simulink model "controller_sdfp_host"  (Simulink 7.3)
settings: Solver=ode45  StartTime=0.0  StopTime=2  RelTol=1e-3
values from neighbouring files (symbols this model uses):
  d = 16    [one_bit_control.m]
  delay_shift1 = -k_preint    (= 0)    [one_bit_control.m]
  delay_shift2 = -k_preint    (= 0)    [one_bit_control.m]
  delay_shift3 = -k_preint    (= 0)    [one_bit_control.m]
  fixpt_adder_in_bitwidth = w    (= 24)    [one_bit_control.m]
  fixpt_adder_in_position = d    (= 16)    [one_bit_control.m]
  fixpt_adder_out_bitwidth = w    (= 24)    [one_bit_control.m]
  fixpt_adder_out_position = d    (= 16)    [one_bit_control.m]
  fixpt_gain_bitwidth = w    (= 24)    [one_bit_control.m]
  fixpt_gain_position = d    (= 16)    [one_bit_control.m]
  k = 2^k_bitshift    (= 0.000244140625)    [one_bit_control.m]
  p0 = 1326*T^3*k^-3    [one_bit_control.m]
  p1 = 9397*T^2*k^-2    [one_bit_control.m]
  p2 = 262.3*T*k^-1    [one_bit_control.m]
  p3 = 16.65    [one_bit_control.m]
  postint_gain1 = k_postint    (= -12)    [one_bit_control.m]
  postint_gain2 = k_postint    (= -12)    [one_bit_control.m]
  postint_gain3 = k_postint    (= -12)    [one_bit_control.m]
  preint_gain1 = k_preint    (= 0)    [one_bit_control.m]
  preint_gain2 = k_preint    (= 0)    [one_bit_control.m]
  preint_gain3 = k_preint    (= 0)    [one_bit_control.m]
  q0 = 0*T^3*k^-3    [one_bit_control.m]
  q1 = 400.8*T^2*k^-2    [one_bit_control.m]
  q2 = 33.2*T*k^-1    [one_bit_control.m]
  T = ts    [one_bit_control.m]
  ts = 1/Fs    [one_bit_control.m]
  w = 24    [one_bit_control.m]
libraries: simulink x16, commnoisgen2 x1, cstblocks x1
(part 1 of 2)
settings Model: Creator=Joseph Poverelli  LastModifiedBy=kunal
settings OptimizationCC: InitFltsAndDblsToZero=on

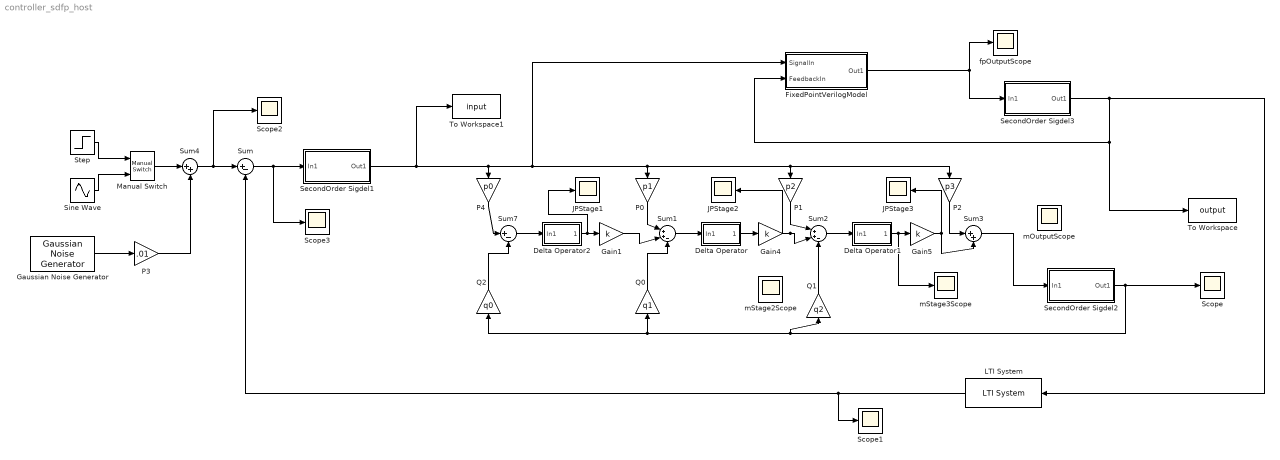
== system controller_sdfp_host ==
  Delta Operator : Subsystem
  Delta Operator1 : Subsystem
  Delta Operator2 : Subsystem
  FixedPointVerilogModel : Subsystem
  Gain1 : Gain  Gain=k  ParameterDataType=sfix(16)  ParameterScaling=2^0  OutDataType=fixdt(1,w,d)  RndMeth=Nearest
  Gain4 : Gain  Gain=k  ParameterDataType=sfix(16)  ParameterScaling=2^0  OutDataType=fixdt(1,w,d)  RndMeth=Nearest
  Gain5 : Gain  Gain=k  ParameterDataType=sfix(16)  ParameterScaling=2^0  OutDataType=fixdt(1,w,d)  RndMeth=Nearest
  Gaussian Noise Generator : commnoisgen2/Gaussian Noise Generator  SystemSampleTime=-1  m=0  d=1  s=41  Ts=T  frameBased=off  sampPerFrame=1  orient=off  outDataType=double
  JPStage1 : Scope
      settings: YMin=-30  YMax=30  SaveName=ScopeData12
  JPStage2 : Scope
      settings: YMin=-0.03  YMax=0.11  SaveName=ScopeData5
  JPStage3 : Scope
      settings: YMin=-0.35  YMax=0.25  SaveName=ScopeData9
  LTI System : cstblocks/LTI System  SystemSampleTime=-1  sys=P  IC=[]
  Manual Switch : simulink/Signal Routing/Manual Switch  SystemSampleTime=-1  sw=0  action=0  varsize=off
  P0 : Gain  Gain=p1  ParameterDataType=sfix(16)  ParameterScaling=2^0  OutDataType=sfix(16)  OutScaling=2^0
  P1 : Gain  Gain=p2  ParameterDataType=sfix(16)  ParameterScaling=2^0  OutDataType=sfix(16)  OutScaling=2^0
  P2 : Gain  Gain=p3  ParameterDataType=sfix(16)  ParameterScaling=2^0  OutDataType=sfix(16)  OutScaling=2^0
  P3 : Gain  Gain=.01  ParameterDataType=sfix(16)  ParameterScaling=2^0  OutDataType=sfix(16)  OutScaling=2^0
  P4 : Gain  Gain=p0  ParameterDataType=sfix(16)  ParameterScaling=2^0  OutDataType=sfix(16)  OutScaling=2^0
  Q0 : Gain  Gain=q1  ParameterDataType=sfix(16)  ParameterScaling=2^0  OutDataType=sfix(16)  OutScaling=2^0
  Q1 : Gain  Gain=q2  ParameterDataType=sfix(16)  ParameterScaling=2^0  OutDataType=sfix(16)  OutScaling=2^0
  Q2 : Gain  Gain=q0  ParameterDataType=sfix(16)  ParameterScaling=2^0  OutDataType=sfix(16)  OutScaling=2^0
  Scope{,1..3} (4 alike) : Scope
      Scope settings: YMin=-1  YMax=1  SaveName=Y  DataFormat=Structure  SampleInput=on  SampleTime=ts
      Scope1 settings: YMin=-0.10575  YMax=-0.1035  SaveName=plant_output  DataFormat=Structure  SampleInput=on  SampleTime=ts
      Scope2 settings: YMin=-0.04  YMax=0.07  SaveName=in  DataFormat=Structure  SampleInput=on  SampleTime=ts
      Scope3 settings: YMin=0.06375  YMax=0.06575  SaveName=error  DataFormat=Array  SampleInput=on  SampleTime=ts
  SecondOrder Sigdel1 : Subsystem
  SecondOrder Sigdel2 : Subsystem
  SecondOrder Sigdel3 : Subsystem
  Sine Wave : Sin  Amplitude=.03  Bias=0  Frequency=2*pi*20  Phase=0  Samples=10  SampleTime=0  Offset=0
  Step : Step  After=.1  SampleTime=ts
  Sum : Sum  Inputs=|+-  OutDataType=sfix(16)  OutScaling=2^0
  Sum1 : Sum  Inputs=|++-  OutDataType=fixdt(1,w,d)  RndMeth=Nearest
  Sum2 : Sum  Inputs=|++-  OutDataType=fixdt(1,w,d)  RndMeth=Nearest
  Sum3 : Sum  Inputs=|++  OutMin=[-p2]  OutMax=[p2]  OutDataType=fixdt(1,w,d)  RndMeth=Nearest  SaturateOnIntegerOverflow=on
  Sum4 : Sum  Inputs=|++  OutDataType=sfix(16)  OutScaling=2^0
  Sum7 : Sum  Inputs=|+-  OutDataType=fixdt(1,w,d)  RndMeth=Nearest
  To Workspace : ToWorkspace  VariableName=output  SampleTime=-1  SaveFormat=Array
  To Workspace1 : ToWorkspace  VariableName=input  SampleTime=-1  SaveFormat=Array
  fpOutputScope : Scope
      settings: YMin=-9.97  YMax=-9.8  SaveName=c_output1  DataFormat=Structure  SampleInput=on  SampleTime=ts
  mOutputScope : Scope
      settings: YMin=-9.97  YMax=-9.8  SaveName=c_output  DataFormat=Structure  SampleInput=on  SampleTime=ts
  mStage2Scope : Scope
      settings: YMin=-0.175  YMax=0.025  SaveName=delta3  DataFormat=Array  SampleInput=on  SampleTime=ts
  mStage3Scope : Scope
      settings: YMin=-0.225  YMax=0.025  SaveName=delta  DataFormat=Array  SampleInput=on  SampleTime=ts
  wires:
  Sum/1 -> SecondOrder Sigdel1/1(In1), Scope3/1
  LTI System/1 -> Sum/2, Scope1/1
  SecondOrder Sigdel1/1(Out1) -> P4/1, P0/1, P1/1, P2/1, FixedPointVerilogModel/1(SignalIn), To Workspace1/1
  Sum3/1 -> SecondOrder Sigdel2/1(In1)
  P0/1 -> Sum1/1
  Q1/1 -> Sum2/3
  P1/1 -> Sum2/1
  P2/1 -> Sum3/1
  Gain5/1 -> Sum3/2, JPStage3/1
  SecondOrder Sigdel2/1(Out1) -> Scope/1, Q1/1, Q0/1, Q2/1
  Delta Operator/1(Out1) -> Gain4/1
  Sum1/1 -> Delta Operator/1(In1)
  Sum2/1 -> Delta Operator1/1(In1)
  Delta Operator1/1(Out1) -> Gain5/1, mStage3Scope/1
  Manual Switch/1 -> Sum4/1
  Gaussian Noise Generator/1 -> P3/1
  Sum4/1 -> Sum/1, Scope2/1
  P3/1 -> Sum4/2
  Sine Wave/1 -> Manual Switch/2
  Step/1 -> Manual Switch/1
  P4/1 -> Sum7/1
  Q2/1 -> Sum7/2
  Delta Operator2/1(Out1) -> Gain1/1, JPStage1/1
  Sum7/1 -> Delta Operator2/1(In1)
  Q0/1 -> Sum1/3
  Gain1/1 -> Sum1/2
  Gain4/1 -> Sum2/2, JPStage2/1
  FixedPointVerilogModel/1(Out1) -> fpOutputScope/1, SecondOrder Sigdel3/1(In1)
  SecondOrder Sigdel3/1(Out1) -> LTI System/1, FixedPointVerilogModel/2(FeedbackIn), To Workspace/1

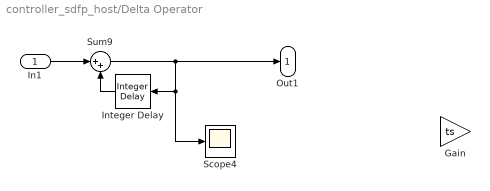
== system controller_sdfp_host/Delta Operator ==
  In1 : Inport  OutDataType=sfix(16)  OutScaling=2^0
  Gain : Gain  Gain=ts  ParameterDataType=sfix(16)  ParameterScaling=2^0  OutDataType=fixdt(1,w,d)  RndMeth=Nearest
  Integer Delay : simulink/Discrete/Integer Delay  vinit=0.0  samptime=-1  NumDelays=1
  Scope4 : Scope
      settings: YMin=-10  YMax=10  SaveName=delta1  DataFormat=Array  SampleInput=on  SampleTime=ts
  Sum9 : Sum  Inputs=|++  OutDataType=fixdt(1,w,d)  RndMeth=Nearest  SampleTime=ts
  Out1 : Outport  OutDataType=sfix(16)  OutScaling=2^0
  wires:
  In1/1 -> Sum9/1
  Sum9/1 -> Integer Delay/1, Scope4/1, Out1/1
  Integer Delay/1 -> Sum9/2

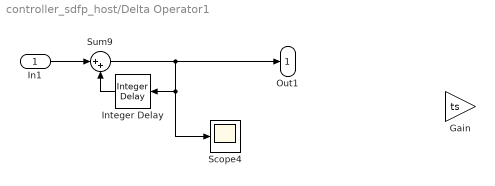
== system controller_sdfp_host/Delta Operator1 ==
  In1 : Inport  OutDataType=sfix(16)  OutScaling=2^0
  Gain : Gain  Gain=ts  ParameterDataType=sfix(16)  ParameterScaling=2^0  OutDataType=fixdt(1,w,d)  RndMeth=Nearest
  Integer Delay : simulink/Discrete/Integer Delay  vinit=0.0  samptime=-1  NumDelays=1
  Scope4 : Scope
      settings: YMin=-10  YMax=10  SaveName=delta2  DataFormat=Array  SampleInput=on  SampleTime=ts
  Sum9 : Sum  Inputs=|++  OutDataType=fixdt(1,w,d)  RndMeth=Nearest  SampleTime=ts
  Out1 : Outport  OutDataType=sfix(16)  OutScaling=2^0
  wires:
  In1/1 -> Sum9/1
  Sum9/1 -> Integer Delay/1, Scope4/1, Out1/1
  Integer Delay/1 -> Sum9/2

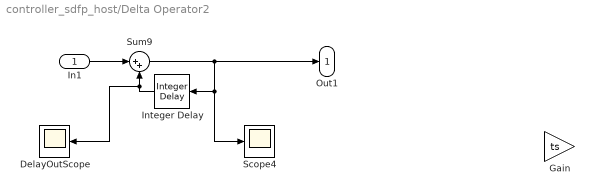
== system controller_sdfp_host/Delta Operator2 ==
  In1 : Inport  OutDataType=sfix(16)  OutScaling=2^0
  DelayOutScope : Scope
      settings: YMin=-900  YMax=700  SaveName=delta4  DataFormat=Array  SampleInput=on  SampleTime=ts
  Gain : Gain  Gain=ts  ParameterDataType=sfix(16)  ParameterScaling=2^0  OutDataType=fixdt(1,w,d)  RndMeth=Nearest
  Integer Delay : simulink/Discrete/Integer Delay  vinit=0.0  samptime=-1  NumDelays=1
  Scope4 : Scope
      settings: TimeRange=0.5  YMin=0.038443  YMax=0.0424896  SaveName=delta43  DataFormat=Array  SampleInput=on  SampleTime=ts
  Sum9 : Sum  Inputs=|++  OutDataType=fixdt(1,w,d)  RndMeth=Nearest  SampleTime=ts
  Out1 : Outport  OutDataType=sfix(16)  OutScaling=2^0
  wires:
  In1/1 -> Sum9/1
  Sum9/1 -> Integer Delay/1, Scope4/1, Out1/1
  Integer Delay/1 -> Sum9/2, DelayOutScope/1

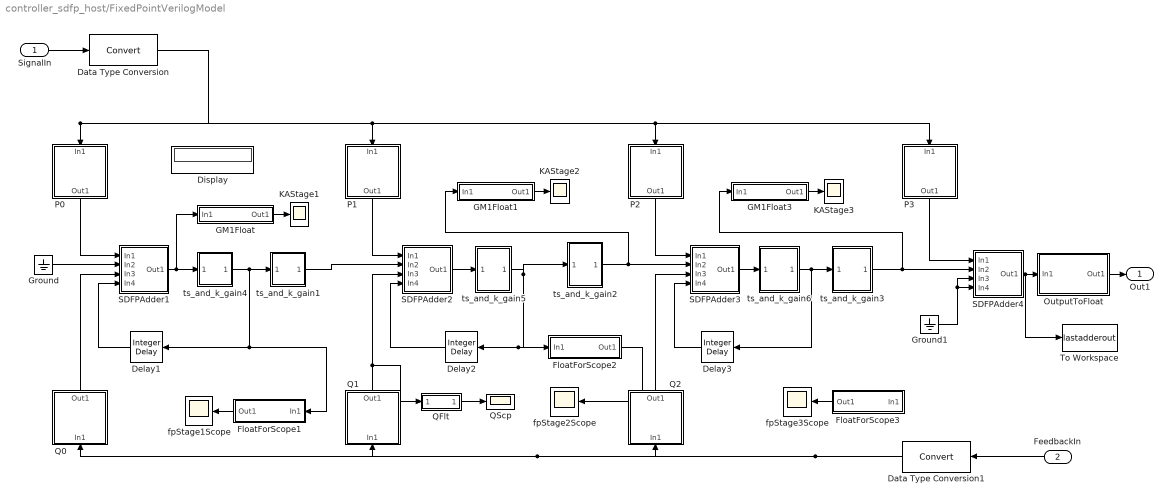
== system controller_sdfp_host/FixedPointVerilogModel ==
  SignalIn : Inport  OutDataType=fixdt(1, 16)  OutScaling=2^0
  FeedbackIn : Inport  Port=2  OutDataType=fixdt(1, 16)  OutScaling=2^0
  Data Type Conversion : DataTypeConversion  OutDataType=fixdt(1, 16)  OutScaling=2^0
  Data Type Conversion1 : DataTypeConversion  OutDataType=fixdt(1, 16)  OutScaling=2^0
  Delay1 : simulink/Discrete/Integer Delay  vinit=0.0  samptime=-1  NumDelays=1
  Delay2 : simulink/Discrete/Integer Delay  vinit=0.0  samptime=-1  NumDelays=1
  Delay3 : simulink/Discrete/Integer Delay  vinit=0.0  samptime=-1  NumDelays=1
  Display : Display
      settings: Format=hex (Stored Integer)
  FloatForScope1 : Subsystem  mask{bitwidth=fixpt_adder_out_bitwidth, fp_position=fixpt_adder_out_position}
      mask prompts: bitwidth "Input Bitwidth"; fp_position "Input Point Position"
      mask Display: disp('Fixed -> Float');
  FloatForScope2 : Subsystem  mask{bitwidth=fixpt_adder_out_bitwidth, fp_position=fixpt_adder_out_position}
      mask prompts: bitwidth "Input Bitwidth"; fp_position "Input Point Position"
      mask Display: disp('Fixed -> Float');
  FloatForScope3 : Subsystem  mask{bitwidth=fixpt_adder_out_bitwidth, fp_position=fixpt_adder_out_position}
      mask prompts: bitwidth "Input Bitwidth"; fp_position "Input Point Position"
      mask Display: disp('Fixed -> Float');
  GM1Float : Subsystem  mask{bitwidth=fixpt_gain_bitwidth, fp_position=fixpt_gain_position}
      mask prompts: bitwidth "Input Bitwidth"; fp_position "Input Point Position"
      mask Display: disp('Fixed -> Float');
  GM1Float1 : Subsystem  mask{bitwidth=fixpt_gain_bitwidth, fp_position=fixpt_gain_position}
      mask prompts: bitwidth "Input Bitwidth"; fp_position "Input Point Position"
      mask Display: disp('Fixed -> Float');
  GM1Float3 : Subsystem  mask{bitwidth=fixpt_gain_bitwidth, fp_position=fixpt_gain_position}
      mask prompts: bitwidth "Input Bitwidth"; fp_position "Input Point Position"
      mask Display: disp('Fixed -> Float');
  Ground : Ground
  Ground1 : Ground
  KAStage1 : Scope
      settings: YMin=-1  YMax=1  SaveName=ScopeData6
  KAStage2 : Scope
      settings: YMin=-0.035  YMax=0.055  SaveName=ScopeData3
  KAStage3 : Scope
      settings: YMin=-0.0007  YMax=0.0009  SaveName=ScopeData14
  OutputToFloat : Subsystem  mask{bitwidth=fixpt_adder_out_bitwidth, fp_position=fixpt_adder_out_position}
      mask prompts: bitwidth "Input Bitwidth"; fp_position "Input Point Position"
      mask Display: disp('Fixed -> Float');
  P0 : Subsystem  mask{gain=p0, bitwidth=fixpt_gain_bitwidth, fp_position=fixpt_gain_position}
      mask prompts: bitwidth "Output Bitwidth"; fp_position "Output Point Position"
      mask Display: plot([0.2 0.9 0.2 0.2],[0 .5 1 0]);disp('GainMux')
  P1 : Subsystem  mask{gain=p1, bitwidth=fixpt_gain_bitwidth, fp_position=fixpt_gain_position}
      mask prompts: bitwidth "Output Bitwidth"; fp_position "Output Point Position"
      mask Display: plot([0.2 0.9 0.2 0.2],[0 .5 1 0]);disp('GainMux')
  P2 : Subsystem  mask{gain=p2, bitwidth=fixpt_gain_bitwidth, fp_position=fixpt_gain_position}
      mask prompts: bitwidth "Output Bitwidth"; fp_position "Output Point Position"
      mask Display: plot([0.2 0.9 0.2 0.2],[0 .5 1 0]);disp('GainMux')
  P3 : Subsystem  mask{gain=p3, bitwidth=fixpt_gain_bitwidth, fp_position=fixpt_gain_position}
      mask prompts: bitwidth "Output Bitwidth"; fp_position "Output Point Position"
      mask Display: plot([0.2 0.9 0.2 0.2],[0 .5 1 0]);disp('GainMux')
  Q0 : Subsystem  mask{gain=q0, bitwidth=fixpt_gain_bitwidth, fp_position=fixpt_gain_position}
      mask prompts: bitwidth "Output Bitwidth"; fp_position "Output Point Position"
      mask Display: plot([0.2 0.9 0.2 0.2],[0 .5 1 0]);disp('GainMux')
  Q1 : Subsystem  mask{gain=q1, bitwidth=fixpt_gain_bitwidth, fp_position=fixpt_gain_position}
      mask prompts: bitwidth "Output Bitwidth"; fp_position "Output Point Position"
      mask Display: plot([0.2 0.9 0.2 0.2],[0 .5 1 0]);disp('GainMux')
  Q2 : Subsystem  mask{gain=q2, bitwidth=fixpt_gain_bitwidth, fp_position=fixpt_gain_position}
      mask prompts: bitwidth "Output Bitwidth"; fp_position "Output Point Position"
      mask Display: plot([0.2 0.9 0.2 0.2],[0 .5 1 0]);disp('GainMux')
  QFlt : Subsystem  mask{bitwidth=fixpt_gain_bitwidth, fp_position=fixpt_gain_position}
      mask prompts: bitwidth "Input Bitwidth"; fp_position "Input Point Position"
      mask Display: disp('Fixed -> Float');
  QScp : Scope
      settings: SaveName=ScopeData11
  SDFPAdder1 : Subsystem  mask{in_bitwidth=fixpt_adder_in_bitwidth, in_fp_position=fixpt_adder_in_position, out_bitwidth=fixpt_adder_out_bitwidth, out_fp_position=fixpt_adder_out_position, in1_shift=0, in2_shift=0, in3_shift=0, in4_shift=delay_shift1}
      mask prompts: in_bitwidth "Input Bitwidth"; in_fp_position "Input Point Position"; out_bitwidth "Output Bitwidth"; out_fp_position "Output Point Position"; in1_shift "Input1 Pre-Shift"; in2_shift "Input2 Pre-Shift"; in3_shift "Input3 Pre-Shift"; in4_shift "Input4 Pre-Shift"
      mask Display: disp(['+\nSDFP'])
  SDFPAdder2 : Subsystem  mask{in_bitwidth=fixpt_adder_in_bitwidth, in_fp_position=fixpt_adder_in_position, out_bitwidth=fixpt_adder_out_bitwidth, out_fp_position=fixpt_adder_out_position, in1_shift=0, in2_shift=0, in3_shift=0, in4_shift=delay_shift2}
      mask prompts: in_bitwidth "Input Bitwidth"; in_fp_position "Input Point Position"; out_bitwidth "Output Bitwidth"; out_fp_position "Output Point Position"; in1_shift "Input1 Pre-Shift"; in2_shift "Input2 Pre-Shift"; in3_shift "Input3 Pre-Shift"; in4_shift "Input4 Pre-Shift"
      mask Display: disp(['+\nSDFP'])
  SDFPAdder3 : Subsystem  mask{in_bitwidth=fixpt_adder_in_bitwidth, in_fp_position=fixpt_adder_in_position, out_bitwidth=fixpt_adder_out_bitwidth, out_fp_position=fixpt_adder_out_position, in1_shift=0, in2_shift=0, in3_shift=0, in4_shift=delay_shift3}
      mask prompts: in_bitwidth "Input Bitwidth"; in_fp_position "Input Point Position"; out_bitwidth "Output Bitwidth"; out_fp_position "Output Point Position"; in1_shift "Input1 Pre-Shift"; in2_shift "Input2 Pre-Shift"; in3_shift "Input3 Pre-Shift"; in4_shift "Input4 Pre-Shift"
      mask Display: disp(['+\nSDFP'])
  SDFPAdder4 : Subsystem  mask{in_bitwidth=fixpt_adder_in_bitwidth, in_fp_position=fixpt_adder_in_position, out_bitwidth=fixpt_adder_out_bitwidth, out_fp_position=fixpt_adder_out_position, in1_shift=0, in2_shift=0, in3_shift=0, in4_shift=0}
      mask prompts: in_bitwidth "Input Bitwidth"; in_fp_position "Input Point Position"; out_bitwidth "Output Bitwidth"; out_fp_position "Output Point Position"; in1_shift "Input1 Pre-Shift"; in2_shift "Input2 Pre-Shift"; in3_shift "Input3 Pre-Shift"; in4_shift "Input4 Pre-Shift"
      mask Display: disp(['+\nSDFP'])
  To Workspace : ToWorkspace  VariableName=lastadderout  SampleTime=-1  SaveFormat=Array
  fpStage1Scope : Scope
      settings: YMin=-800  YMax=700
  fpStage2Scope : Scope
      settings: YMin=0  YMax=275
  fpStage3Scope : Scope
      settings: YMin=0  YMax=275  SaveName=ScopeData2
  ts_and_k_gain1 : Subsystem  mask{shift_amount=postint_gain1}
      mask init:
      | if(shift_amount > 0)
      |     dispval=sprintf('<< %d',shift_amount);
      | else
      |     dispval=sprintf('>> %d',-shift_amount);
      | end
      mask Display: disp(dispval);
  ts_and_k_gain2 : Subsystem  mask{shift_amount=postint_gain2}
      mask init:
      | if(shift_amount > 0)
      |     dispval=sprintf('<< %d',shift_amount);
      | else
      |     dispval=sprintf('>> %d',-shift_amount);
      | end
      mask Display: disp(dispval);
  ts_and_k_gain3 : Subsystem  mask{shift_amount=postint_gain3}
      mask init:
      | if(shift_amount > 0)
      |     dispval=sprintf('<< %d',shift_amount);
      | else
      |     dispval=sprintf('>> %d',-shift_amount);
      | end
      mask Display: disp(dispval);
  ts_and_k_gain4 : Subsystem  mask{shift_amount=preint_gain1}
      mask init:
      | if(shift_amount > 0)
      |     dispval=sprintf('<< %d',shift_amount);
      | else
      |     dispval=sprintf('>> %d',-shift_amount);
      | end
      mask Display: disp(dispval);
  ts_and_k_gain5 : Subsystem  mask{shift_amount=preint_gain2}
      mask init:
      | if(shift_amount > 0)
      |     dispval=sprintf('<< %d',shift_amount);
      | else
      |     dispval=sprintf('>> %d',-shift_amount);
      | end
      mask Display: disp(dispval);
  ts_and_k_gain6 : Subsystem  mask{shift_amount=preint_gain3}
      mask init:
      | if(shift_amount > 0)
      |     dispval=sprintf('<< %d',shift_amount);
      | else
      |     dispval=sprintf('>> %d',-shift_amount);
      | end
      mask Display: disp(dispval);
  Out1 : Outport  OutDataType=fixdt(1, 16)  OutScaling=2^0
  wires:
  P0/1(Out1) -> SDFPAdder1/1(In1)
  Ground/1 -> SDFPAdder1/2(In2)
  Delay1/1 -> SDFPAdder1/4(In4)
  Q0/1(Out1) -> SDFPAdder1/3(In3)
  P1/1(Out1) -> SDFPAdder2/1(In1)
  Delay2/1 -> SDFPAdder2/4(In4)
  Q1/1(Out1) -> QFlt/1(In1), SDFPAdder2/3(In3)
  SDFPAdder2/1(Out1) -> ts_and_k_gain5/1(In1)
  ts_and_k_gain1/1(Out1) -> SDFPAdder2/2(In2)
  P2/1(Out1) -> SDFPAdder3/1(In1)
  Delay3/1 -> SDFPAdder3/4(In4)
  Q2/1(Out1) -> SDFPAdder3/3(In3)
  ts_and_k_gain2/1(Out1) -> SDFPAdder3/2(In2), GM1Float1/1(In1)
  FeedbackIn/1 -> Data Type Conversion1/1
  ts_and_k_gain3/1(Out1) -> SDFPAdder4/2(In2), GM1Float3/1(In1)
  P3/1(Out1) -> SDFPAdder4/1(In1)
  SDFPAdder4/1(Out1) -> OutputToFloat/1(In1), To Workspace/1
  SignalIn/1 -> Data Type Conversion/1
  Data Type Conversion/1 -> P0/1(In1), P1/1(In1), P2/1(In1), P3/1(In1)
  Data Type Conversion1/1 -> Q2/1(In1), Q1/1(In1), Q0/1(In1)
  FloatForScope2/1(Out1) -> fpStage2Scope/1
  OutputToFloat/1(Out1) -> Out1/1
  QFlt/1(Out1) -> QScp/1
  GM1Float/1(Out1) -> KAStage1/1
  Ground1/1 -> SDFPAdder4/3(In3), SDFPAdder4/4(In4)
  FloatForScope1/1(Out1) -> fpStage1Scope/1
  SDFPAdder1/1(Out1) -> ts_and_k_gain4/1(In1), GM1Float/1(In1)
  ts_and_k_gain5/1(Out1) -> Delay2/1, FloatForScope2/1(In1), ts_and_k_gain2/1(In1)
  FloatForScope3/1(Out1) -> fpStage3Scope/1
  SDFPAdder3/1(Out1) -> ts_and_k_gain6/1(In1)
  ts_and_k_gain6/1(Out1) -> ts_and_k_gain3/1(In1), Delay3/1
  ts_and_k_gain4/1(Out1) -> ts_and_k_gain1/1(In1), Delay1/1, FloatForScope1/1(In1)
  GM1Float1/1(Out1) -> KAStage2/1
  GM1Float3/1(Out1) -> KAStage3/1

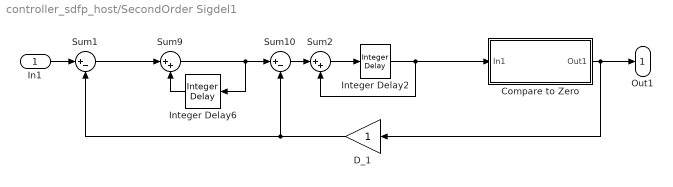
== system controller_sdfp_host/SecondOrder Sigdel1 ==
  In1 : Inport  OutDataType=sfix(16)  OutScaling=2^0
  Compare to Zero : Subsystem
  D_1 : Gain  ParameterDataType=sfix(16)  ParameterScaling=2^0  OutDataType=sfix(16)  OutScaling=2^0  SampleTime=ts
  Integer Delay2 : simulink/Discrete/Integer Delay  vinit=0.0  samptime=-1  NumDelays=1
  Integer Delay6 : simulink/Discrete/Integer Delay  vinit=0.0  samptime=-1  NumDelays=1
  Sum1 : Sum  Inputs=|+-  OutDataType=sfix(16)  OutScaling=2^0  SampleTime=ts
  Sum10 : Sum  Inputs=|+-  OutDataType=sfix(16)  OutScaling=2^0
  Sum2 : Sum  Inputs=|++  OutDataType=sfix(16)  OutScaling=2^0
  Sum9 : Sum  Inputs=|++  OutDataType=sfix(16)  OutScaling=2^0  SampleTime=ts
  Out1 : Outport  OutDataType=sfix(16)  OutScaling=2^0
  wires:
  Sum1/1 -> Sum9/1
  In1/1 -> Sum1/1
  Compare to Zero/1(Out1) -> D_1/1, Out1/1
  Sum2/1 -> Integer Delay2/1
  Integer Delay2/1 -> Sum2/2, Compare to Zero/1(In1)
  Sum9/1 -> Integer Delay6/1, Sum10/1
  Integer Delay6/1 -> Sum9/2
  Sum10/1 -> Sum2/1
  D_1/1 -> Sum1/2, Sum10/2

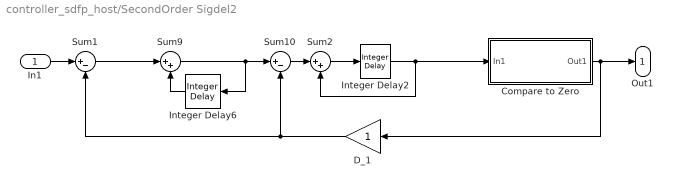
== system controller_sdfp_host/SecondOrder Sigdel2 ==
  In1 : Inport  OutDataType=sfix(16)  OutScaling=2^0
  Compare to Zero : Subsystem
  D_1 : Gain  ParameterDataType=sfix(16)  ParameterScaling=2^0  OutDataType=sfix(16)  OutScaling=2^0  SampleTime=ts
  Integer Delay2 : simulink/Discrete/Integer Delay  vinit=0.0  samptime=-1  NumDelays=1
  Integer Delay6 : simulink/Discrete/Integer Delay  vinit=0.0  samptime=-1  NumDelays=1
  Sum1 : Sum  Inputs=|+-  OutDataType=sfix(16)  OutScaling=2^0  SampleTime=ts
  Sum10 : Sum  Inputs=|+-  OutDataType=sfix(16)  OutScaling=2^0
  Sum2 : Sum  Inputs=|++  OutDataType=sfix(16)  OutScaling=2^0
  Sum9 : Sum  Inputs=|++  OutDataType=sfix(16)  OutScaling=2^0  SampleTime=ts
  Out1 : Outport  OutDataType=sfix(16)  OutScaling=2^0
  wires:
  Sum1/1 -> Sum9/1
  In1/1 -> Sum1/1
  Compare to Zero/1(Out1) -> D_1/1, Out1/1
  Sum2/1 -> Integer Delay2/1
  Integer Delay2/1 -> Sum2/2, Compare to Zero/1(In1)
  Sum9/1 -> Integer Delay6/1, Sum10/1
  Integer Delay6/1 -> Sum9/2
  Sum10/1 -> Sum2/1
  D_1/1 -> Sum1/2, Sum10/2

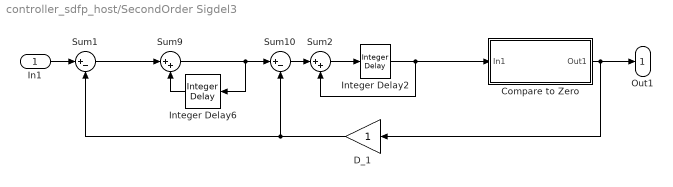
== system controller_sdfp_host/SecondOrder Sigdel3 ==
  In1 : Inport  OutDataType=sfix(16)  OutScaling=2^0
  Compare to Zero : Subsystem
  D_1 : Gain  ParameterDataType=sfix(16)  ParameterScaling=2^0  OutDataType=sfix(16)  OutScaling=2^0  SampleTime=ts
  Integer Delay2 : simulink/Discrete/Integer Delay  vinit=0.0  samptime=-1  NumDelays=1
  Integer Delay6 : simulink/Discrete/Integer Delay  vinit=0.0  samptime=-1  NumDelays=1
  Sum1 : Sum  Inputs=|+-  OutDataType=sfix(16)  OutScaling=2^0  SampleTime=ts
  Sum10 : Sum  Inputs=|+-  OutDataType=sfix(16)  OutScaling=2^0
  Sum2 : Sum  Inputs=|++  OutDataType=sfix(16)  OutScaling=2^0
  Sum9 : Sum  Inputs=|++  OutDataType=sfix(16)  OutScaling=2^0  SampleTime=ts
  Out1 : Outport  OutDataType=sfix(16)  OutScaling=2^0
  wires:
  Sum1/1 -> Sum9/1
  In1/1 -> Sum1/1
  Compare to Zero/1(Out1) -> D_1/1, Out1/1
  Sum2/1 -> Integer Delay2/1
  Integer Delay2/1 -> Sum2/2, Compare to Zero/1(In1)
  Sum9/1 -> Integer Delay6/1, Sum10/1
  Integer Delay6/1 -> Sum9/2
  Sum10/1 -> Sum2/1
  D_1/1 -> Sum1/2, Sum10/2

== system controller_sdfp_host/FixedPointVerilogModel/FloatForScope1 ==
  In1 : Inport  OutDataType=fixdt(1, 16)  OutScaling=2^0
  S-Function Builder : S-Function  InitFcn=try, set_param(gcb,'FunctionName','SDFPFromFixed'), end  FunctionName=SDFPFromFixed  Parameters=uint32(bitwidth),uint32(fp_position)  SFunctionModules=SDFPFromFixed_wrapper fpconv  WizardData=DataTag0  EnableBusSupport=off  mask(S-Function Builder){}
      mask help: The S-Function Builder block creates a wrapper C-MEX S-function from your supplied C code with multiple input ports, output ports, and a variable number of scalar, vector, or matrix parameters. The input and output ports can propagate Simulink built-in data types, fixed-point datatypes, complex, frame, 1-D, and 2-D signals. This block also supports discrete and continuous states of type real. You can optionally have the block generate a TLC file to be used with Real-Time Workshop for code generation.
      mask init:
      | val = [[.9  0.75 0.75 1 1 .9 .9 1]',[1 1 0.75 0.75 .9 .9 1 .9]'];try , sys = get_param(gcb,'SfunBuilderFcnName');if isempty(sys), sys = get_param(gcb,'FunctionName'); end,catch, sys = get_param(gcb,'FunctionName'); end
      settings: CopyFcn=set_param(gcbh,'LinkStatus','none')  PreSaveFcn=try, set_param(gcb,'FunctionName','SDFPFromFixed'), end  OpenFcn=sfunctionwizard(gcbh)
      mask Display: plot(val(:,1),val(:,2)),disp(sys)port_label('input',1,'fixed_in')port_label('output',1,'float_out')
  Out1 : Outport  OutDataType=fixdt(1, 16)  OutScaling=2^0
  wires:
  S-Function Builder/1 -> Out1/1
  In1/1 -> S-Function Builder/1

== system controller_sdfp_host/FixedPointVerilogModel/FloatForScope2 ==
  In1 : Inport  OutDataType=fixdt(1, 16)  OutScaling=2^0
  S-Function Builder : S-Function  InitFcn=try, set_param(gcb,'FunctionName','SDFPFromFixed'), end  FunctionName=SDFPFromFixed  Parameters=uint32(bitwidth),uint32(fp_position)  SFunctionModules=SDFPFromFixed_wrapper fpconv  WizardData=DataTag1  EnableBusSupport=off  mask(S-Function Builder){}
      mask help: The S-Function Builder block creates a wrapper C-MEX S-function from your supplied C code with multiple input ports, output ports, and a variable number of scalar, vector, or matrix parameters. The input and output ports can propagate Simulink built-in data types, fixed-point datatypes, complex, frame, 1-D, and 2-D signals. This block also supports discrete and continuous states of type real. You can optionally have the block generate a TLC file to be used with Real-Time Workshop for code generation.
      mask init: same as controller_sdfp_host/FixedPointVerilogModel/FloatForScope1/S-Function Builder
      settings: CopyFcn=set_param(gcbh,'LinkStatus','none')  PreSaveFcn=try, set_param(gcb,'FunctionName','SDFPFromFixed'), end  OpenFcn=sfunctionwizard(gcbh)
      mask Display: plot(val(:,1),val(:,2)),disp(sys)port_label('input',1,'fixed_in')port_label('output',1,'float_out')
  Out1 : Outport  OutDataType=fixdt(1, 16)  OutScaling=2^0
  wires:
  In1/1 -> S-Function Builder/1
  S-Function Builder/1 -> Out1/1

== system controller_sdfp_host/FixedPointVerilogModel/FloatForScope3 ==
  In1 : Inport  OutDataType=fixdt(1, 16)  OutScaling=2^0
  S-Function Builder : S-Function  InitFcn=try, set_param(gcb,'FunctionName','SDFPFromFixed'), end  FunctionName=SDFPFromFixed  Parameters=uint32(bitwidth),uint32(fp_position)  SFunctionModules=SDFPFromFixed_wrapper fpconv  WizardData=DataTag2  EnableBusSupport=off  mask(S-Function Builder){}
      mask help: The S-Function Builder block creates a wrapper C-MEX S-function from your supplied C code with multiple input ports, output ports, and a variable number of scalar, vector, or matrix parameters. The input and output ports can propagate Simulink built-in data types, fixed-point datatypes, complex, frame, 1-D, and 2-D signals. This block also supports discrete and continuous states of type real. You can optionally have the block generate a TLC file to be used with Real-Time Workshop for code generation.
      mask init: same as controller_sdfp_host/FixedPointVerilogModel/FloatForScope1/S-Function Builder
      settings: CopyFcn=set_param(gcbh,'LinkStatus','none')  PreSaveFcn=try, set_param(gcb,'FunctionName','SDFPFromFixed'), end  OpenFcn=sfunctionwizard(gcbh)
      mask Display: plot(val(:,1),val(:,2)),disp(sys)port_label('input',1,'fixed_in')port_label('output',1,'float_out')
  Out1 : Outport  OutDataType=fixdt(1, 16)  OutScaling=2^0
  wires:
  S-Function Builder/1 -> Out1/1
  In1/1 -> S-Function Builder/1

== system controller_sdfp_host/FixedPointVerilogModel/GM1Float ==
  In1 : Inport  OutDataType=fixdt(1, 16)  OutScaling=2^0
  S-Function Builder : S-Function  InitFcn=try, set_param(gcb,'FunctionName','SDFPFromFixed'), end  FunctionName=SDFPFromFixed  Parameters=uint32(bitwidth),uint32(fp_position)  SFunctionModules=SDFPFromFixed_wrapper fpconv  WizardData=DataTag3  EnableBusSupport=off  mask(S-Function Builder){}
      mask help: The S-Function Builder block creates a wrapper C-MEX S-function from your supplied C code with multiple input ports, output ports, and a variable number of scalar, vector, or matrix parameters. The input and output ports can propagate Simulink built-in data types, fixed-point datatypes, complex, frame, 1-D, and 2-D signals. This block also supports discrete and continuous states of type real. You can optionally have the block generate a TLC file to be used with Real-Time Workshop for code generation.
      mask init: same as controller_sdfp_host/FixedPointVerilogModel/FloatForScope1/S-Function Builder
      settings: CopyFcn=set_param(gcbh,'LinkStatus','none')  PreSaveFcn=try, set_param(gcb,'FunctionName','SDFPFromFixed'), end  OpenFcn=sfunctionwizard(gcbh)
      mask Display: plot(val(:,1),val(:,2)),disp(sys)port_label('input',1,'fixed_in')port_label('output',1,'float_out')
  Out1 : Outport  OutDataType=fixdt(1, 16)  OutScaling=2^0
  wires:
  In1/1 -> S-Function Builder/1
  S-Function Builder/1 -> Out1/1

== system controller_sdfp_host/FixedPointVerilogModel/GM1Float1 ==
  In1 : Inport  OutDataType=fixdt(1, 16)  OutScaling=2^0
  S-Function Builder : S-Function  InitFcn=try, set_param(gcb,'FunctionName','SDFPFromFixed'), end  FunctionName=SDFPFromFixed  Parameters=uint32(bitwidth),uint32(fp_position)  SFunctionModules=SDFPFromFixed_wrapper fpconv  WizardData=DataTag4  EnableBusSupport=off  mask(S-Function Builder){}
      mask help: The S-Function Builder block creates a wrapper C-MEX S-function from your supplied C code with multiple input ports, output ports, and a variable number of scalar, vector, or matrix parameters. The input and output ports can propagate Simulink built-in data types, fixed-point datatypes, complex, frame, 1-D, and 2-D signals. This block also supports discrete and continuous states of type real. You can optionally have the block generate a TLC file to be used with Real-Time Workshop for code generation.
      mask init: same as controller_sdfp_host/FixedPointVerilogModel/FloatForScope1/S-Function Builder
      settings: CopyFcn=set_param(gcbh,'LinkStatus','none')  PreSaveFcn=try, set_param(gcb,'FunctionName','SDFPFromFixed'), end  OpenFcn=sfunctionwizard(gcbh)
      mask Display: plot(val(:,1),val(:,2)),disp(sys)port_label('input',1,'fixed_in')port_label('output',1,'float_out')
  Out1 : Outport  OutDataType=fixdt(1, 16)  OutScaling=2^0
  wires:
  In1/1 -> S-Function Builder/1
  S-Function Builder/1 -> Out1/1

== system controller_sdfp_host/FixedPointVerilogModel/GM1Float3 ==
  In1 : Inport  OutDataType=fixdt(1, 16)  OutScaling=2^0
  S-Function Builder : S-Function  InitFcn=try, set_param(gcb,'FunctionName','SDFPFromFixed'), end  FunctionName=SDFPFromFixed  Parameters=uint32(bitwidth),uint32(fp_position)  SFunctionModules=SDFPFromFixed_wrapper fpconv  WizardData=DataTag5  EnableBusSupport=off  mask(S-Function Builder){}
      mask help: The S-Function Builder block creates a wrapper C-MEX S-function from your supplied C code with multiple input ports, output ports, and a variable number of scalar, vector, or matrix parameters. The input and output ports can propagate Simulink built-in data types, fixed-point datatypes, complex, frame, 1-D, and 2-D signals. This block also supports discrete and continuous states of type real. You can optionally have the block generate a TLC file to be used with Real-Time Workshop for code generation.
      mask init: same as controller_sdfp_host/FixedPointVerilogModel/FloatForScope1/S-Function Builder
      settings: CopyFcn=set_param(gcbh,'LinkStatus','none')  PreSaveFcn=try, set_param(gcb,'FunctionName','SDFPFromFixed'), end  OpenFcn=sfunctionwizard(gcbh)
      mask Display: plot(val(:,1),val(:,2)),disp(sys)port_label('input',1,'fixed_in')port_label('output',1,'float_out')
  Out1 : Outport  OutDataType=fixdt(1, 16)  OutScaling=2^0
  wires:
  In1/1 -> S-Function Builder/1
  S-Function Builder/1 -> Out1/1

== system controller_sdfp_host/FixedPointVerilogModel/OutputToFloat ==
  In1 : Inport  OutDataType=fixdt(1, 16)  OutScaling=2^0
  S-Function Builder : S-Function  InitFcn=try, set_param(gcb,'FunctionName','SDFPFromFixed'), end  FunctionName=SDFPFromFixed  Parameters=uint32(bitwidth),uint32(fp_position)  SFunctionModules=SDFPFromFixed_wrapper fpconv  WizardData=DataTag6  EnableBusSupport=off  mask(S-Function Builder){}
      mask help: The S-Function Builder block creates a wrapper C-MEX S-function from your supplied C code with multiple input ports, output ports, and a variable number of scalar, vector, or matrix parameters. The input and output ports can propagate Simulink built-in data types, fixed-point datatypes, complex, frame, 1-D, and 2-D signals. This block also supports discrete and continuous states of type real. You can optionally have the block generate a TLC file to be used with Real-Time Workshop for code generation.
      mask init: same as controller_sdfp_host/FixedPointVerilogModel/FloatForScope1/S-Function Builder
      settings: CopyFcn=set_param(gcbh,'LinkStatus','none')  PreSaveFcn=try, set_param(gcb,'FunctionName','SDFPFromFixed'), end  OpenFcn=sfunctionwizard(gcbh)
      mask Display: plot(val(:,1),val(:,2)),disp(sys)port_label('input',1,'fixed_in')port_label('output',1,'float_out')
  Out1 : Outport  OutDataType=fixdt(1, 16)  OutScaling=2^0
  wires:
  S-Function Builder/1 -> Out1/1
  In1/1 -> S-Function Builder/1

== system controller_sdfp_host/FixedPointVerilogModel/P0 ==
  In1 : Inport  OutDataType=fixdt(1, 16)  OutScaling=2^0
  S-Function Builder : S-Function  InitFcn=try, set_param(gcb,'FunctionName','SDFPGainSwitch'), end  FunctionName=SDFPGainSwitch  Parameters=single(gain),uint32(bitwidth),uint32(fp_position)  SFunctionModules=SDFPGainSwitch_wrapper fpconv  WizardData=DataTag7  EnableBusSupport=off  mask(S-Function Builder){}
      mask help: The S-Function Builder block creates a wrapper C-MEX S-function from your supplied C code with multiple input ports, output ports, and a variable number of scalar, vector, or matrix parameters. The input and output ports can propagate Simulink built-in data types, fixed-point datatypes, complex, frame, 1-D, and 2-D signals. This block also supports discrete and continuous states of type real. You can optionally have the block generate a TLC file to be used with Real-Time Workshop for code generation.
      mask init: same as controller_sdfp_host/FixedPointVerilogModel/FloatForScope1/S-Function Builder
      settings: CopyFcn=set_param(gcbh,'LinkStatus','none')  PreSaveFcn=try, set_param(gcb,'FunctionName','SDFPGainSwitch'), end  OpenFcn=sfunctionwizard(gcbh)
      mask Display: plot(val(:,1),val(:,2)),disp(sys)port_label('input',1,'sd_in')port_label('output',1,'gain_out')port_label('output',2,'fixpt_out')port_label('output',3,'p_gain_out')
  Out1 : Outport  OutDataType=fixdt(1, 16)  OutScaling=2^0
  wires:
  S-Function Builder/1 -> Out1/1
  In1/1 -> S-Function Builder/1

== system controller_sdfp_host/FixedPointVerilogModel/P1 ==
  In1 : Inport  OutDataType=fixdt(1, 16)  OutScaling=2^0
  Display : Display
      settings: Format=hex (Stored Integer)  Decimation=32
  S-Function Builder : S-Function  InitFcn=try, set_param(gcb,'FunctionName','SDFPGainSwitch'), end  FunctionName=SDFPGainSwitch  Parameters=single(gain),uint32(bitwidth),uint32(fp_position)  SFunctionModules=SDFPGainSwitch_wrapper fpconv  WizardData=DataTag8  EnableBusSupport=off  mask(S-Function Builder){}
      mask help: The S-Function Builder block creates a wrapper C-MEX S-function from your supplied C code with multiple input ports, output ports, and a variable number of scalar, vector, or matrix parameters. The input and output ports can propagate Simulink built-in data types, fixed-point datatypes, complex, frame, 1-D, and 2-D signals. This block also supports discrete and continuous states of type real. You can optionally have the block generate a TLC file to be used with Real-Time Workshop for code generation.
      mask init: same as controller_sdfp_host/FixedPointVerilogModel/FloatForScope1/S-Function Builder
      settings: CopyFcn=set_param(gcbh,'LinkStatus','none')  PreSaveFcn=try, set_param(gcb,'FunctionName','SDFPGainSwitch'), end  OpenFcn=sfunctionwizard(gcbh)
      mask Display: plot(val(:,1),val(:,2)),disp(sys)port_label('input',1,'sd_in')port_label('output',1,'gain_out')port_label('output',2,'fixpt_out')port_label('output',3,'p_gain_out')
  Out1 : Outport  OutDataType=fixdt(1, 16)  OutScaling=2^0
  wires:
  In1/1 -> S-Function Builder/1
  S-Function Builder/1 -> Out1/1
  S-Function Builder/2 -> Display/1

== system controller_sdfp_host/FixedPointVerilogModel/P2 ==
  In1 : Inport  OutDataType=fixdt(1, 16)  OutScaling=2^0
  Display : Display
      settings: Format=hex (Stored Integer)  Decimation=32
  S-Function Builder : S-Function  InitFcn=try, set_param(gcb,'FunctionName','SDFPGainSwitch'), end  FunctionName=SDFPGainSwitch  Parameters=single(gain),uint32(bitwidth),uint32(fp_position)  SFunctionModules=SDFPGainSwitch_wrapper fpconv  WizardData=DataTag9  EnableBusSupport=off  mask(S-Function Builder){}
      mask help: The S-Function Builder block creates a wrapper C-MEX S-function from your supplied C code with multiple input ports, output ports, and a variable number of scalar, vector, or matrix parameters. The input and output ports can propagate Simulink built-in data types, fixed-point datatypes, complex, frame, 1-D, and 2-D signals. This block also supports discrete and continuous states of type real. You can optionally have the block generate a TLC file to be used with Real-Time Workshop for code generation.
      mask init: same as controller_sdfp_host/FixedPointVerilogModel/FloatForScope1/S-Function Builder
      settings: CopyFcn=set_param(gcbh,'LinkStatus','none')  PreSaveFcn=try, set_param(gcb,'FunctionName','SDFPGainSwitch'), end  OpenFcn=sfunctionwizard(gcbh)
      mask Display: plot(val(:,1),val(:,2)),disp(sys)port_label('input',1,'sd_in')port_label('output',1,'gain_out')port_label('output',2,'fixpt_out')port_label('output',3,'p_gain_out')
  Out1 : Outport  OutDataType=fixdt(1, 16)  OutScaling=2^0
  wires:
  S-Function Builder/1 -> Out1/1
  In1/1 -> S-Function Builder/1
  S-Function Builder/2 -> Display/1

== system controller_sdfp_host/FixedPointVerilogModel/P3 ==
  In1 : Inport  OutDataType=fixdt(1, 16)  OutScaling=2^0
  S-Function Builder : S-Function  InitFcn=try, set_param(gcb,'FunctionName','SDFPGainSwitch'), end  FunctionName=SDFPGainSwitch  Parameters=single(gain),uint32(bitwidth),uint32(fp_position)  SFunctionModules=SDFPGainSwitch_wrapper fpconv  EnableBusSupport=off  mask(S-Function Builder){}
      mask help: The S-Function Builder block creates a wrapper C-MEX S-function from your supplied C code with multiple input ports, output ports, and a variable number of scalar, vector, or matrix parameters. The input and output ports can propagate Simulink built-in data types, fixed-point datatypes, complex, frame, 1-D, and 2-D signals. This block also supports discrete and continuous states of type real. You can optionally have the block generate a TLC file to be used with Real-Time Workshop for code generation.
      mask init: same as controller_sdfp_host/FixedPointVerilogModel/FloatForScope1/S-Function Builder
      settings: CopyFcn=set_param(gcbh,'LinkStatus','none')  PreSaveFcn=try, set_param(gcb,'FunctionName','SDFPGainSwitch'), end  OpenFcn=sfunctionwizard(gcbh)
      mask Display: plot(val(:,1),val(:,2)),disp(sys)port_label('input',1,'sd_in')port_label('output',1,'gain_out')
  Out1 : Outport  OutDataType=fixdt(1, 16)  OutScaling=2^0
  wires:
  S-Function Builder/1 -> Out1/1
  In1/1 -> S-Function Builder/1

== system controller_sdfp_host/FixedPointVerilogModel/Q0 ==
  In1 : Inport  OutDataType=fixdt(1, 16)  OutScaling=2^0
  S-Function Builder : S-Function  InitFcn=try, set_param(gcb,'FunctionName','SDFPGainSwitch'), end  FunctionName=SDFPGainSwitch  Parameters=single(gain),uint32(bitwidth),uint32(fp_position)  SFunctionModules=SDFPGainSwitch_wrapper fpconv  WizardData=DataTag10  EnableBusSupport=off  mask(S-Function Builder){}
      mask help: The S-Function Builder block creates a wrapper C-MEX S-function from your supplied C code with multiple input ports, output ports, and a variable number of scalar, vector, or matrix parameters. The input and output ports can propagate Simulink built-in data types, fixed-point datatypes, complex, frame, 1-D, and 2-D signals. This block also supports discrete and continuous states of type real. You can optionally have the block generate a TLC file to be used with Real-Time Workshop for code generation.
      mask init: same as controller_sdfp_host/FixedPointVerilogModel/FloatForScope1/S-Function Builder
      settings: CopyFcn=set_param(gcbh,'LinkStatus','none')  PreSaveFcn=try, set_param(gcb,'FunctionName','SDFPGainSwitch'), end  OpenFcn=sfunctionwizard(gcbh)
      mask Display: plot(val(:,1),val(:,2)),disp(sys)port_label('input',1,'sd_in')port_label('output',1,'gain_out')
  Out1 : Outport  OutDataType=fixdt(1, 16)  OutScaling=2^0
  wires:
  In1/1 -> S-Function Builder/1
  S-Function Builder/1 -> Out1/1

== system controller_sdfp_host/FixedPointVerilogModel/Q1 ==
  In1 : Inport  OutDataType=fixdt(1, 16)  OutScaling=2^0
  S-Function Builder : S-Function  InitFcn=try, set_param(gcb,'FunctionName','SDFPGainSwitch'), end  FunctionName=SDFPGainSwitch  Parameters=single(gain),uint32(bitwidth),uint32(fp_position)  SFunctionModules=SDFPGainSwitch_wrapper fpconv  EnableBusSupport=off  mask(S-Function Builder){}
      mask help: The S-Function Builder block creates a wrapper C-MEX S-function from your supplied C code with multiple input ports, output ports, and a variable number of scalar, vector, or matrix parameters. The input and output ports can propagate Simulink built-in data types, fixed-point datatypes, complex, frame, 1-D, and 2-D signals. This block also supports discrete and continuous states of type real. You can optionally have the block generate a TLC file to be used with Real-Time Workshop for code generation.
      mask init: same as controller_sdfp_host/FixedPointVerilogModel/FloatForScope1/S-Function Builder
      settings: CopyFcn=set_param(gcbh,'LinkStatus','none')  PreSaveFcn=try, set_param(gcb,'FunctionName','SDFPGainSwitch'), end  OpenFcn=sfunctionwizard(gcbh)
      mask Display: plot(val(:,1),val(:,2)),disp(sys)port_label('input',1,'sd_in')port_label('output',1,'gain_out')
  Out1 : Outport  OutDataType=fixdt(1, 16)  OutScaling=2^0
  wires:
  S-Function Builder/1 -> Out1/1
  In1/1 -> S-Function Builder/1

== system controller_sdfp_host/FixedPointVerilogModel/Q2 ==
  In1 : Inport  OutDataType=fixdt(1, 16)  OutScaling=2^0
  S-Function Builder : S-Function  InitFcn=try, set_param(gcb,'FunctionName','SDFPGainSwitch'), end  FunctionName=SDFPGainSwitch  Parameters=single(gain),uint32(bitwidth),uint32(fp_position)  SFunctionModules=SDFPGainSwitch_wrapper fpconv  WizardData=DataTag11  EnableBusSupport=off  mask(S-Function Builder){}
      mask help: The S-Function Builder block creates a wrapper C-MEX S-function from your supplied C code with multiple input ports, output ports, and a variable number of scalar, vector, or matrix parameters. The input and output ports can propagate Simulink built-in data types, fixed-point datatypes, complex, frame, 1-D, and 2-D signals. This block also supports discrete and continuous states of type real. You can optionally have the block generate a TLC file to be used with Real-Time Workshop for code generation.
      mask init: same as controller_sdfp_host/FixedPointVerilogModel/FloatForScope1/S-Function Builder
      settings: CopyFcn=set_param(gcbh,'LinkStatus','none')  PreSaveFcn=try, set_param(gcb,'FunctionName','SDFPGainSwitch'), end  OpenFcn=sfunctionwizard(gcbh)
      mask Display: plot(val(:,1),val(:,2)),disp(sys)port_label('input',1,'sd_in')port_label('output',1,'gain_out')
  Out1 : Outport  OutDataType=fixdt(1, 16)  OutScaling=2^0
  wires:
  In1/1 -> S-Function Builder/1
  S-Function Builder/1 -> Out1/1

== system controller_sdfp_host/FixedPointVerilogModel/QFlt ==
  In1 : Inport  OutDataType=fixdt(1, 16)  OutScaling=2^0
  S-Function Builder : S-Function  InitFcn=try, set_param(gcb,'FunctionName','SDFPFromFixed'), end  FunctionName=SDFPFromFixed  Parameters=uint32(bitwidth),uint32(fp_position)  SFunctionModules=SDFPFromFixed_wrapper fpconv  WizardData=DataTag12  EnableBusSupport=off  mask(S-Function Builder){}
      mask help: The S-Function Builder block creates a wrapper C-MEX S-function from your supplied C code with multiple input ports, output ports, and a variable number of scalar, vector, or matrix parameters. The input and output ports can propagate Simulink built-in data types, fixed-point datatypes, complex, frame, 1-D, and 2-D signals. This block also supports discrete and continuous states of type real. You can optionally have the block generate a TLC file to be used with Real-Time Workshop for code generation.
      mask init: same as controller_sdfp_host/FixedPointVerilogModel/FloatForScope1/S-Function Builder
      settings: CopyFcn=set_param(gcbh,'LinkStatus','none')  PreSaveFcn=try, set_param(gcb,'FunctionName','SDFPFromFixed'), end  OpenFcn=sfunctionwizard(gcbh)
      mask Display: plot(val(:,1),val(:,2)),disp(sys)port_label('input',1,'fixed_in')port_label('output',1,'float_out')
  Out1 : Outport  OutDataType=fixdt(1, 16)  OutScaling=2^0
  wires:
  In1/1 -> S-Function Builder/1
  S-Function Builder/1 -> Out1/1

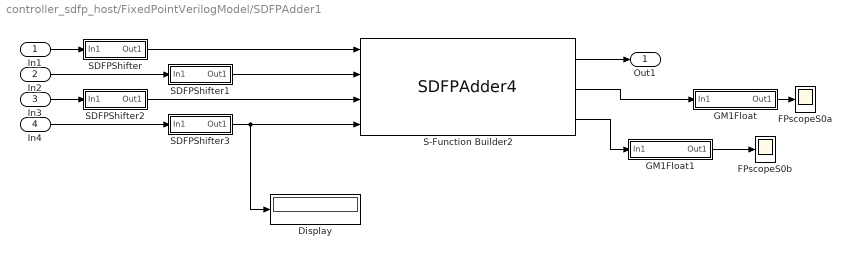
== system controller_sdfp_host/FixedPointVerilogModel/SDFPAdder1 ==
  In1 : Inport  OutDataType=fixdt(1, 16)  OutScaling=2^0
  In2 : Inport  Port=2  OutDataType=fixdt(1, 16)  OutScaling=2^0
  In3 : Inport  Port=3  OutDataType=fixdt(1, 16)  OutScaling=2^0
  In4 : Inport  Port=4  OutDataType=fixdt(1, 16)  OutScaling=2^0
  Display : Display
      settings: Format=hex (Stored Integer)
  FPscopeS0a : Scope
      settings: TimeRange=0.03999999999999998  YMin=-0.1  YMax=0.1  SaveName=ScopeData15
  FPscopeS0b : Scope
      settings: SaveName=ScopeData16
  GM1Float : Subsystem  mask{bitwidth=fixpt_gain_bitwidth, fp_position=fixpt_gain_position}
      mask prompts: bitwidth "Input Bitwidth"; fp_position "Input Point Position"
      mask Display: disp('Fixed -> Float');
  GM1Float1 : Subsystem  mask{bitwidth=fixpt_gain_bitwidth, fp_position=fixpt_gain_position}
      mask prompts: bitwidth "Input Bitwidth"; fp_position "Input Point Position"
      mask Display: disp('Fixed -> Float');
  S-Function Builder2 : S-Function  InitFcn=try, set_param(gcb,'FunctionName','SDFPAdder4'), end  FunctionName=SDFPAdder4  Parameters=uint32(in_bitwidth),uint32(in_fp_position),uint32(out_bitwidth),uint32(out_fp_position)  SFunctionModules=SDFPAdder4_wrapper  WizardData=DataTag15  EnableBusSupport=off  mask(S-Function Builder){}
      mask help: The S-Function Builder block creates a wrapper C-MEX S-function from your supplied C code with multiple input ports, output ports, and a variable number of scalar, vector, or matrix parameters. The input and output ports can propagate Simulink built-in data types, fixed-point datatypes, complex, frame, 1-D, and 2-D signals. This block also supports discrete and continuous states of type real. You can optionally have the block generate a TLC file to be used with Real-Time Workshop for code generation.
      mask init: same as controller_sdfp_host/FixedPointVerilogModel/FloatForScope1/S-Function Builder
      settings: CopyFcn=set_param(gcbh,'LinkStatus','none')  PreSaveFcn=try, set_param(gcb,'FunctionName','SDFPAdder4'), end  OpenFcn=sfunctionwizard(gcbh)
      mask Display: plot(val(:,1),val(:,2)),disp(sys)port_label('input',1,'in0')port_label('input',2,'in1')port_label('input',3,'in2')port_label('input',4,'in3')port_label('output',1,'adder_out')port_label('output',2,'DBG_in01')port_label('output',3,'DBG_in012')
  SDFPShifter : Subsystem  mask{shift_amount=in1_shift}
      mask init:
      | if(shift_amount > 0)
      |     dispval=sprintf('<< %d',shift_amount);
      | else
      |     dispval=sprintf('>> %d',-shift_amount);
      | end
      mask Display: disp(dispval);
  SDFPShifter1 : Subsystem  mask{shift_amount=in2_shift}
      mask init:
      | if(shift_amount > 0)
      |     dispval=sprintf('<< %d',shift_amount);
      | else
      |     dispval=sprintf('>> %d',-shift_amount);
      | end
      mask Display: disp(dispval);
  SDFPShifter2 : Subsystem  mask{shift_amount=in3_shift}
      mask init:
      | if(shift_amount > 0)
      |     dispval=sprintf('<< %d',shift_amount);
      | else
      |     dispval=sprintf('>> %d',-shift_amount);
      | end
      mask Display: disp(dispval);
  SDFPShifter3 : Subsystem  mask{shift_amount=in4_shift}
      mask init:
      | if(shift_amount > 0)
      |     dispval=sprintf('<< %d',shift_amount);
      | else
      |     dispval=sprintf('>> %d',-shift_amount);
      | end
      mask Display: disp(dispval);
  Out1 : Outport  OutDataType=fixdt(1, 16)  OutScaling=2^0
  wires:
  In1/1 -> SDFPShifter/1(In1)
  In2/1 -> SDFPShifter1/1(In1)
  In3/1 -> SDFPShifter2/1(In1)
  In4/1 -> SDFPShifter3/1(In1)
  S-Function Builder2/1 -> Out1/1
  GM1Float/1(Out1) -> FPscopeS0a/1
  S-Function Builder2/2 -> GM1Float/1(In1)
  GM1Float1/1(Out1) -> FPscopeS0b/1
  S-Function Builder2/3 -> GM1Float1/1(In1)
  SDFPShifter/1(Out1) -> S-Function Builder2/1
  SDFPShifter1/1(Out1) -> S-Function Builder2/2
  SDFPShifter2/1(Out1) -> S-Function Builder2/3
  SDFPShifter3/1(Out1) -> S-Function Builder2/4, Display/1
